simulink model "M10B39_es_V1"  (R2024b)
settings: Solver=ode23tb  StartTime=0.0  StopTime=20  FixedStep=0.001  RelTol=1e-3  EnableMultiTasking=on
InitFcn:
  | initAll;
values from neighbouring files (symbols this model uses):
  acom = 100    [initAll_V1.m]    (also in initAll_V2.m; initAll_V3.m; parameterinit.mat)
  AVm0 = [4.26082678503 4.656135219]    [parameterinit.mat]
  bcom = 50    [initAll_V1.m]    (also in initAll_V2.m; initAll_V3.m; parameterinit.mat)
  commun = 0*commun    [initAll_V1.m]    (also in initAll_V2.m; initAll_V3.m; parameterinit.mat = [0  0  0; 0  0  0; 0  0  0; 0  0  0])
  DataDelay = 0.0*DataDelay    [initAll_V1.m]    (also in initAll_V2.m; initAll_V3.m; parameterinit.mat = [0  0  0; 0  0  0; 0  0  0; 0  0  0])
  ESinit =     [parameterinit.mat]
  fB = 50    [initAll.m]    (also in initAll_V1.m; initAll_V2.m; initAll_V3.m; parameterinit.mat)
  Geninit = Generator_init(opdata,SynMach_in_gidx)    [initAll.m]    (also in initAll_V1.m; initAll_V2.m; initAll_V3.m = Generator_init(opdata_all,SynMach_in_gidx1); parameterinit.mat = )
  lam = 100    [initAll_V1.m]    (also in initAll_V2.m; initAll_V3.m; parameterinit.mat)
  SgridB = 100    [initAll.m]    (also in initAll_V1.m; initAll_V2.m; initAll_V3.m; parameterinit.mat)
  wB = 2*pi*fB    (= 314.159265359)    [initAll.m]    (also in initAll_V1.m; initAll_V2.m; initAll_V3.m; parameterinit.mat)
  Windinit =     [parameterinit.mat]
  YY_load = [3.65450097002 -2.05705688056 0 0 0 0 0 0 0 0 0 0 ... (1521 elements, 39x39)]    [parameterinit.mat]    (also in powerflowcaculate.m = full(YY))
undefined symbols (not defined in the file or in its folder): c1, c2, c3, c4, c5, c6, cp_nom, lambda_nom, P_wind_base, Pelec_base, Pnom
libraries: spsBistableLib x12, simulink_extras x4, slpidlib x1, simulink x1
(part 7 of 7)

== system M10B39_es_V1/Genrators/Wind Generator - DFIG1/Asynchronous Machine Equations /3th order Transient Equations ==
  note: Comparison of 5th order and 3rd order machine models for doubly fed induction generator (DFIG) wind turbines
      | //J.B. Ekanayake a,c, * , L. Holdsworth b , N. Jenkins b,c
  Isxy : Inport
  Vrxy : Inport  Port=2
  s / ω_B : Inport  Port=3
  Trip : Inport  Port=4
  Add : Sum  Inputs=+-
  Add1 : Sum  Inputs=-+
  Add2 : Sum  Inputs=+-
  Add3 : Sum  Inputs=--
  Constant1 : Constant  Value=0
  Constant2 : Constant  Value=0
  Demux : Demux  Outputs=2
  Demux1 : Demux  Outputs=2
  Demux2 : Demux  Outputs=2
  Ex : Integrator  InitialCondition=Ex0
  Ey : Integrator  InitialCondition=Ey0
  Fcn : Fcn  Expr=u(2)-(Xa-Xa1)*u(1)
  Fcn1 : Fcn  Expr=u(2)+(Xa-Xa1)*u(1)
  Gain{,1,6,8} (4 alike) : Gain  Gain=Lm/Lr
  Gain2 : Gain  Gain=1/Ta0
  Gain3 : Gain  Gain=1/Ta0
  Gain5 : Gain  Gain=1/Lm
  Gain7 : Gain  Gain=1/Lm
  Multiply : Product
  Multiply1 : Product  Inputs=3
  Multiply2 : Product
  Multiply3 : Product  Inputs=3
  Mux{,1..3} (4 alike) : Mux  Inputs=2
  Sum : Sum  Inputs=|+-
  Sum1 : Sum  Inputs=|+-
  Switch{1..4} (4 alike) : Switch  Criteria=u2 ~= 0  Threshold=0.5  InputSameDT=off
  Irxy : Outport
  Eyx : Outport  Port=2
  wires:
  [Trip] -> Switch4/2, Switch1/2
  Constant2/1 -> Switch4/1, Switch1/1
  Switch4/1 -> Mux/2, [Ey], Mux2/1
  Ey/1 -> Switch4/3  "Ey"
  Switch1/1 -> Ey/1
  Sum/1 -> Switch1/3
  [Trip] -> Switch2/2, Switch3/2
  Constant1/1 -> Switch3/1, Switch2/1
  Switch3/1 -> Mux1/2, [Ex], Mux2/2
  Ex/1 -> Switch3/3  "Ex"
  Sum1/1 -> Switch2/3
  Switch2/1 -> Ex/1
  Trip/1 -> [Trip]
  [Vry] -> Gain8/1
  Gain8/1 -> Multiply2/1
  Gain/1 -> Multiply/1
  Add3/1 -> [Iry]
  [Isy] -> Gain1/1
  Add2/1 -> [Irx]
  Gain1/1 -> Add3/2
  [Isx] -> Gain6/1
  [Ey] -> Gain5/1
  Gain7/1 -> Add3/1
  [Ex] -> Gain7/1
  Gain6/1 -> Add2/2
  Gain5/1 -> Add2/1
  [Irx] -> Mux3/1
  [Iry] -> Mux3/2
  Mux3/1 -> Irxy/1
  Gain2/1 -> Sum/2
  Gain3/1 -> Sum1/2
  Mux2/1 -> Eyx/1
  Fcn1/1 -> Gain3/1
  Mux1/1 -> Fcn1/1
  [Isy] -> Mux1/1
  Add1/1 -> Sum1/1
  Multiply2/1 -> Add1/1
  Multiply3/1 -> Add1/2
  [s] -> Multiply3/1
  [Ey] -> Multiply3/3
  [w_b] -> Multiply3/2
  [w_b] -> Multiply2/2
  Multiply1/1 -> Add/2
  Add/1 -> Sum/1
  Multiply/1 -> Add/1
  Fcn/1 -> Gain2/1
  Mux/1 -> Fcn/1
  [Isx] -> Mux/1
  [Ex] -> Multiply1/3
  [w_b] -> Multiply1/2
  [s] -> Multiply1/1
  [w_b] -> Multiply/2
  [Vrx] -> Gain/1
  Demux1/2 -> [Vry]
  Demux1/1 -> [Vrx]
  Demux2/2 -> [w_b]
  Demux2/1 -> [s]
  s / ω_B/1 -> Demux2/1
  Vrxy/1 -> Demux1/1
  Isxy/1 -> Demux/1
  Demux/2 -> [Isy]
  Demux/1 -> [Isx]

== system M10B39_es_V1/Genrators/Wind Generator - DFIG1/Asynchronous Machine Equations /Interface ==
  delta : Inport
  Eqd : Inport  Port=2
  Add2 : Sum
  Add3 : Sum
  Bx : Constant  Value=Xa1/( Rs^2+Xa1^2 )
  By : Constant  Value=-Xa1/( Rs^2+Xa1^2 )
  Demux1 : Demux  Outputs=2
  Fcn : Fcn  Expr=(Rs*cos(u(1))+Xa1*sin(u(1))) / (Rs^2+Xa1^2)
  Fcn1 : Fcn  Expr=(Rs*cos(u(1))+Xa1*sin(u(1))) / (Rs^2+Xa1^2)
  Fcn2 : Fcn  Expr=(-Rs*sin(u(1))+Xa1*cos(u(1))) / (Rs^2+Xa1^2)
  Fcn3 : Fcn  Expr=(Rs*sin(u(1))-Xa1*cos(u(1))) / (Rs^2+Xa1^2)
  Gx : Constant  Value=Rs/( Rs^2+Xa1^2 )
  Gy : Constant  Value=Rs/( Rs^2+Xa1^2 )
  Mux3 : Mux  Inputs=2
  Mux4 : Mux
  Product{4..7} (4 alike) : Product
  Igxy1 : Outport
  GBxy : Outport  Port=2
  wires:
  Gx/1 -> Mux4/1
  [gx] -> Product4/1
  [Eq] -> Product5/1
  Product7/1 -> Add3/2
  Product4/1 -> Add2/1
  Product5/1 -> Add2/2
  Add3/1 -> [I1y]
  Product6/1 -> Add3/1
  [Eq] -> Product7/1
  [gy] -> Product7/2
  [bx] -> Product5/2
  Add2/1 -> [I1x]
  [Ed] -> Product6/2
  [Ed] -> Product4/2
  [by] -> Product6/1
  Fcn3/1 -> [by]
  Fcn2/1 -> [bx]
  Fcn1/1 -> [gy]
  Fcn/1 -> [gx]
  [delta] -> Fcn/1, Fcn3/1, Fcn2/1, Fcn1/1
  Demux1/2 -> [Ed]
  Demux1/1 -> [Eq]
  Mux4/1 -> GBxy/1
  By/1 -> Mux4/4
  Bx/1 -> Mux4/3
  Gy/1 -> Mux4/2
  Mux3/1 -> Igxy1/1
  [I1y] -> Mux3/2
  [I1x] -> Mux3/1
  Eqd/1 -> Demux1/1
  delta/1 -> [delta]

== system M10B39_es_V1/Genrators/Wind Generator - DFIG1/Rotor Side Converter control/Power Control ==
  note: $P_s^{ref}=2*(0.5000*\omega_r^2+0.0500*\omega_r+0.1200)$
  wr : Inport
  0-inf1 : Saturate  UpperLimit=inf  LowerLimit=0
  Tracking Curve5 : Fcn  Expr=1.162*u(1)^2
  Ps_ref : Outport
  wires:
  Tracking Curve5/1 -> Ps_ref/1
  0-inf1/1 -> Tracking Curve5/1
  wr/1 -> 0-inf1/1

== system M10B39_es_V1/Genrators/Wind Generator - DFIG1/Wind Turbine/Subsystem ==
  wind speed : Inport
  generator speed : Inport  Port=2
  Pitch angle (deg) : Inport  Port=3
  1/cp_nom : Gain  Gain=1/cp_nom  SaturateOnIntegerOverflow=on  OutDataTypeStr=Inherit: Same as input  ParamDataTypeStr=Inherit: Same as input
  Avoid division by zero : Saturate  UpperLimit=1e6  LowerLimit=1e-6
  "Avoid division by zero " : Saturate  UpperLimit=1e6  LowerLimit=1e-6
  Fcn : Fcn  Expr=1/(1/(u[1]+0.08*u[2])-0.035/(u[2]^3+1))
  Fcn1 : Fcn  Expr=c1*(c2/u[2]-c3*u[3]-c4)*exp(-c5/u[2])+c6*u[1]
  Gain : Gain  Gain=-1  SaturateOnIntegerOverflow=on  OutDataTypeStr=Inherit: Same as input  ParamDataTypeStr=Inherit: Same as input
  Mux : Mux  Inputs=2
  Mux1 : Mux  Inputs=3
  Product : Product  Inputs=/*  SaturateOnIntegerOverflow=on  OutDataTypeStr=Inherit: Same as first input
  "Product " : Product  SaturateOnIntegerOverflow=on  OutDataTypeStr=Inherit: Same as first input
  Product1 : Product  Inputs=*/  InputSameDT=on  SaturateOnIntegerOverflow=on  OutDataTypeStr=Inherit: Same as first input
  Saturation1 : Saturate  UpperLimit=inf  LowerLimit=1e-6
  lambda_nom : Gain  Gain=lambda_nom  SaturateOnIntegerOverflow=on  OutDataTypeStr=Inherit: Same as input  ParamDataTypeStr=Inherit: Same as input
  pu->pu : Gain  Gain=P_wind_base*Pnom/Pelec_base  SaturateOnIntegerOverflow=on  OutDataTypeStr=Inherit: Same as input  ParamDataTypeStr=Inherit: Same as input
  wind_speed^3 : Fcn  Expr=u(1)^3
  Tm : Outport
  wires:
  Pitch angle (deg)/1 -> Mux/2, Mux1/3
  Saturation1/1 -> Mux/1, Mux1/1
  Fcn1/1 -> 1/cp_nom/1
  Mux1/1 -> Fcn1/1
  Mux/1 -> Fcn/1
  Fcn/1 -> Mux1/2  "lambda_i"
  Gain/1 -> Tm/1
  Product1/1 -> Gain/1
  "Product "/1 -> pu->pu/1  "Pm_pu"
  lambda_nom/1 -> Saturation1/1
  generator speed/1 -> Avoid division by zero/1, Product/2
  "Avoid division by zero "/1 -> Product/1
  pu->pu/1 -> Product1/1
  Product/1 -> lambda_nom/1
  Avoid division by zero/1 -> Product1/2
  wind_speed^3/1 -> "Product "/1  "Pwind_pu"
  1/cp_nom/1 -> "Product "/2  "cp_pu"
  wind speed/1 -> "Avoid division by zero "/1, wind_speed^3/1  "wind_speed_pu"

== system M10B39_es_V1/Genrators/Wind Generator - DFIG2/Asynchronous Machine Equations /3th order Transient Equations ==
  note: Comparison of 5th order and 3rd order machine models for doubly fed induction generator (DFIG) wind turbines
      | //J.B. Ekanayake a,c, * , L. Holdsworth b , N. Jenkins b,c
  Isxy : Inport
  Vrxy : Inport  Port=2
  s / ω_B : Inport  Port=3
  Trip : Inport  Port=4
  Add : Sum  Inputs=+-
  Add1 : Sum  Inputs=-+
  Add2 : Sum  Inputs=+-
  Add3 : Sum  Inputs=--
  Constant1 : Constant  Value=0
  Constant2 : Constant  Value=0
  Demux : Demux  Outputs=2
  Demux1 : Demux  Outputs=2
  Demux2 : Demux  Outputs=2
  Ex : Integrator  InitialCondition=Ex0
  Ey : Integrator  InitialCondition=Ey0
  Fcn : Fcn  Expr=u(2)-(Xa-Xa1)*u(1)
  Fcn1 : Fcn  Expr=u(2)+(Xa-Xa1)*u(1)
  Gain{,1,6,8} (4 alike) : Gain  Gain=Lm/Lr
  Gain2 : Gain  Gain=1/Ta0
  Gain3 : Gain  Gain=1/Ta0
  Gain5 : Gain  Gain=1/Lm
  Gain7 : Gain  Gain=1/Lm
  Multiply : Product
  Multiply1 : Product  Inputs=3
  Multiply2 : Product
  Multiply3 : Product  Inputs=3
  Mux{,1..3} (4 alike) : Mux  Inputs=2
  Sum : Sum  Inputs=|+-
  Sum1 : Sum  Inputs=|+-
  Switch{1..4} (4 alike) : Switch  Criteria=u2 ~= 0  Threshold=0.5  InputSameDT=off
  Irxy : Outport
  Eyx : Outport  Port=2
  wires:
  [Trip] -> Switch4/2, Switch1/2
  Constant2/1 -> Switch4/1, Switch1/1
  Switch4/1 -> Mux/2, [Ey], Mux2/1
  Ey/1 -> Switch4/3  "Ey"
  Switch1/1 -> Ey/1
  Sum/1 -> Switch1/3
  [Trip] -> Switch2/2, Switch3/2
  Constant1/1 -> Switch3/1, Switch2/1
  Switch3/1 -> Mux1/2, [Ex], Mux2/2
  Ex/1 -> Switch3/3  "Ex"
  Sum1/1 -> Switch2/3
  Switch2/1 -> Ex/1
  Trip/1 -> [Trip]
  [Vry] -> Gain8/1
  Gain8/1 -> Multiply2/1
  Gain/1 -> Multiply/1
  Add3/1 -> [Iry]
  [Isy] -> Gain1/1
  Add2/1 -> [Irx]
  Gain1/1 -> Add3/2
  [Isx] -> Gain6/1
  [Ey] -> Gain5/1
  Gain7/1 -> Add3/1
  [Ex] -> Gain7/1
  Gain6/1 -> Add2/2
  Gain5/1 -> Add2/1
  [Irx] -> Mux3/1
  [Iry] -> Mux3/2
  Mux3/1 -> Irxy/1
  Gain2/1 -> Sum/2
  Gain3/1 -> Sum1/2
  Mux2/1 -> Eyx/1
  Fcn1/1 -> Gain3/1
  Mux1/1 -> Fcn1/1
  [Isy] -> Mux1/1
  Add1/1 -> Sum1/1
  Multiply2/1 -> Add1/1
  Multiply3/1 -> Add1/2
  [s] -> Multiply3/1
  [Ey] -> Multiply3/3
  [w_b] -> Multiply3/2
  [w_b] -> Multiply2/2
  Multiply1/1 -> Add/2
  Add/1 -> Sum/1
  Multiply/1 -> Add/1
  Fcn/1 -> Gain2/1
  Mux/1 -> Fcn/1
  [Isx] -> Mux/1
  [Ex] -> Multiply1/3
  [w_b] -> Multiply1/2
  [s] -> Multiply1/1
  [w_b] -> Multiply/2
  [Vrx] -> Gain/1
  Demux1/2 -> [Vry]
  Demux1/1 -> [Vrx]
  Demux2/2 -> [w_b]
  Demux2/1 -> [s]
  s / ω_B/1 -> Demux2/1
  Vrxy/1 -> Demux1/1
  Isxy/1 -> Demux/1
  Demux/2 -> [Isy]
  Demux/1 -> [Isx]

== system M10B39_es_V1/Genrators/Wind Generator - DFIG2/Asynchronous Machine Equations /Interface ==
  delta : Inport
  Eqd : Inport  Port=2
  Add2 : Sum
  Add3 : Sum
  Bx : Constant  Value=Xa1/( Rs^2+Xa1^2 )
  By : Constant  Value=-Xa1/( Rs^2+Xa1^2 )
  Demux1 : Demux  Outputs=2
  Fcn : Fcn  Expr=(Rs*cos(u(1))+Xa1*sin(u(1))) / (Rs^2+Xa1^2)
  Fcn1 : Fcn  Expr=(Rs*cos(u(1))+Xa1*sin(u(1))) / (Rs^2+Xa1^2)
  Fcn2 : Fcn  Expr=(-Rs*sin(u(1))+Xa1*cos(u(1))) / (Rs^2+Xa1^2)
  Fcn3 : Fcn  Expr=(Rs*sin(u(1))-Xa1*cos(u(1))) / (Rs^2+Xa1^2)
  Gx : Constant  Value=Rs/( Rs^2+Xa1^2 )
  Gy : Constant  Value=Rs/( Rs^2+Xa1^2 )
  Mux3 : Mux  Inputs=2
  Mux4 : Mux
  Product{4..7} (4 alike) : Product
  Igxy1 : Outport
  GBxy : Outport  Port=2
  wires:
  Gx/1 -> Mux4/1
  [gx] -> Product4/1
  [Eq] -> Product5/1
  Product7/1 -> Add3/2
  Product4/1 -> Add2/1
  Product5/1 -> Add2/2
  Add3/1 -> [I1y]
  Product6/1 -> Add3/1
  [Eq] -> Product7/1
  [gy] -> Product7/2
  [bx] -> Product5/2
  Add2/1 -> [I1x]
  [Ed] -> Product6/2
  [Ed] -> Product4/2
  [by] -> Product6/1
  Fcn3/1 -> [by]
  Fcn2/1 -> [bx]
  Fcn1/1 -> [gy]
  Fcn/1 -> [gx]
  [delta] -> Fcn/1, Fcn3/1, Fcn2/1, Fcn1/1
  Demux1/2 -> [Ed]
  Demux1/1 -> [Eq]
  Mux4/1 -> GBxy/1
  By/1 -> Mux4/4
  Bx/1 -> Mux4/3
  Gy/1 -> Mux4/2
  Mux3/1 -> Igxy1/1
  [I1y] -> Mux3/2
  [I1x] -> Mux3/1
  Eqd/1 -> Demux1/1
  delta/1 -> [delta]

== system M10B39_es_V1/Genrators/Wind Generator - DFIG2/Rotor Side Converter control/Power Control ==
  note: $P_s^{ref}=2*(0.5000*\omega_r^2+0.0500*\omega_r+0.1200)$
  wr : Inport
  0-inf1 : Saturate  UpperLimit=inf  LowerLimit=0
  Tracking Curve5 : Fcn  Expr=1.162*u(1)^2
  Ps_ref : Outport
  wires:
  Tracking Curve5/1 -> Ps_ref/1
  0-inf1/1 -> Tracking Curve5/1
  wr/1 -> 0-inf1/1

== system M10B39_es_V1/Genrators/Wind Generator - DFIG2/Wind Turbine/Subsystem ==
  wind speed : Inport
  generator speed : Inport  Port=2
  Pitch angle (deg) : Inport  Port=3
  1/cp_nom : Gain  Gain=1/cp_nom  SaturateOnIntegerOverflow=on  OutDataTypeStr=Inherit: Same as input  ParamDataTypeStr=Inherit: Same as input
  Avoid division by zero : Saturate  UpperLimit=1e6  LowerLimit=1e-6
  "Avoid division by zero " : Saturate  UpperLimit=1e6  LowerLimit=1e-6
  Fcn : Fcn  Expr=1/(1/(u[1]+0.08*u[2])-0.035/(u[2]^3+1))
  Fcn1 : Fcn  Expr=c1*(c2/u[2]-c3*u[3]-c4)*exp(-c5/u[2])+c6*u[1]
  Gain : Gain  Gain=-1  SaturateOnIntegerOverflow=on  OutDataTypeStr=Inherit: Same as input  ParamDataTypeStr=Inherit: Same as input
  Mux : Mux  Inputs=2
  Mux1 : Mux  Inputs=3
  Product : Product  Inputs=/*  SaturateOnIntegerOverflow=on  OutDataTypeStr=Inherit: Same as first input
  "Product " : Product  SaturateOnIntegerOverflow=on  OutDataTypeStr=Inherit: Same as first input
  Product1 : Product  Inputs=*/  InputSameDT=on  SaturateOnIntegerOverflow=on  OutDataTypeStr=Inherit: Same as first input
  Saturation1 : Saturate  UpperLimit=inf  LowerLimit=1e-6
  lambda_nom : Gain  Gain=lambda_nom  SaturateOnIntegerOverflow=on  OutDataTypeStr=Inherit: Same as input  ParamDataTypeStr=Inherit: Same as input
  pu->pu : Gain  Gain=P_wind_base*Pnom/Pelec_base  SaturateOnIntegerOverflow=on  OutDataTypeStr=Inherit: Same as input  ParamDataTypeStr=Inherit: Same as input
  wind_speed^3 : Fcn  Expr=u(1)^3
  Tm : Outport
  wires:
  Pitch angle (deg)/1 -> Mux/2, Mux1/3
  Saturation1/1 -> Mux/1, Mux1/1
  Fcn1/1 -> 1/cp_nom/1
  Mux1/1 -> Fcn1/1
  Mux/1 -> Fcn/1
  Fcn/1 -> Mux1/2  "lambda_i"
  Gain/1 -> Tm/1
  Product1/1 -> Gain/1
  "Product "/1 -> pu->pu/1  "Pm_pu"
  lambda_nom/1 -> Saturation1/1
  generator speed/1 -> Avoid division by zero/1, Product/2
  "Avoid division by zero "/1 -> Product/1
  pu->pu/1 -> Product1/1
  Product/1 -> lambda_nom/1
  Avoid division by zero/1 -> Product1/2
  wind_speed^3/1 -> "Product "/1  "Pwind_pu"
  1/cp_nom/1 -> "Product "/2  "cp_pu"
  wind speed/1 -> "Avoid division by zero "/1, wind_speed^3/1  "wind_speed_pu"

== system M10B39_es_V1/Genrators/Wind Generator - DFIG3/Asynchronous Machine Equations /3th order Transient Equations ==
  note: Comparison of 5th order and 3rd order machine models for doubly fed induction generator (DFIG) wind turbines
      | //J.B. Ekanayake a,c, * , L. Holdsworth b , N. Jenkins b,c
  Isxy : Inport
  Vrxy : Inport  Port=2
  s / ω_B : Inport  Port=3
  Trip : Inport  Port=4
  Add : Sum  Inputs=+-
  Add1 : Sum  Inputs=-+
  Add2 : Sum  Inputs=+-
  Add3 : Sum  Inputs=--
  Constant1 : Constant  Value=0
  Constant2 : Constant  Value=0
  Demux : Demux  Outputs=2
  Demux1 : Demux  Outputs=2
  Demux2 : Demux  Outputs=2
  Ex : Integrator  InitialCondition=Ex0
  Ey : Integrator  InitialCondition=Ey0
  Fcn : Fcn  Expr=u(2)-(Xa-Xa1)*u(1)
  Fcn1 : Fcn  Expr=u(2)+(Xa-Xa1)*u(1)
  Gain{,1,6,8} (4 alike) : Gain  Gain=Lm/Lr
  Gain2 : Gain  Gain=1/Ta0
  Gain3 : Gain  Gain=1/Ta0
  Gain5 : Gain  Gain=1/Lm
  Gain7 : Gain  Gain=1/Lm
  Multiply : Product
  Multiply1 : Product  Inputs=3
  Multiply2 : Product
  Multiply3 : Product  Inputs=3
  Mux{,1..3} (4 alike) : Mux  Inputs=2
  Sum : Sum  Inputs=|+-
  Sum1 : Sum  Inputs=|+-
  Switch{1..4} (4 alike) : Switch  Criteria=u2 ~= 0  Threshold=0.5  InputSameDT=off
  Irxy : Outport
  Eyx : Outport  Port=2
  wires:
  [Trip] -> Switch4/2, Switch1/2
  Constant2/1 -> Switch4/1, Switch1/1
  Switch4/1 -> Mux/2, [Ey], Mux2/1
  Ey/1 -> Switch4/3  "Ey"
  Switch1/1 -> Ey/1
  Sum/1 -> Switch1/3
  [Trip] -> Switch2/2, Switch3/2
  Constant1/1 -> Switch3/1, Switch2/1
  Switch3/1 -> Mux1/2, [Ex], Mux2/2
  Ex/1 -> Switch3/3  "Ex"
  Sum1/1 -> Switch2/3
  Switch2/1 -> Ex/1
  Trip/1 -> [Trip]
  [Vry] -> Gain8/1
  Gain8/1 -> Multiply2/1
  Gain/1 -> Multiply/1
  Add3/1 -> [Iry]
  [Isy] -> Gain1/1
  Add2/1 -> [Irx]
  Gain1/1 -> Add3/2
  [Isx] -> Gain6/1
  [Ey] -> Gain5/1
  Gain7/1 -> Add3/1
  [Ex] -> Gain7/1
  Gain6/1 -> Add2/2
  Gain5/1 -> Add2/1
  [Irx] -> Mux3/1
  [Iry] -> Mux3/2
  Mux3/1 -> Irxy/1
  Gain2/1 -> Sum/2
  Gain3/1 -> Sum1/2
  Mux2/1 -> Eyx/1
  Fcn1/1 -> Gain3/1
  Mux1/1 -> Fcn1/1
  [Isy] -> Mux1/1
  Add1/1 -> Sum1/1
  Multiply2/1 -> Add1/1
  Multiply3/1 -> Add1/2
  [s] -> Multiply3/1
  [Ey] -> Multiply3/3
  [w_b] -> Multiply3/2
  [w_b] -> Multiply2/2
  Multiply1/1 -> Add/2
  Add/1 -> Sum/1
  Multiply/1 -> Add/1
  Fcn/1 -> Gain2/1
  Mux/1 -> Fcn/1
  [Isx] -> Mux/1
  [Ex] -> Multiply1/3
  [w_b] -> Multiply1/2
  [s] -> Multiply1/1
  [w_b] -> Multiply/2
  [Vrx] -> Gain/1
  Demux1/2 -> [Vry]
  Demux1/1 -> [Vrx]
  Demux2/2 -> [w_b]
  Demux2/1 -> [s]
  s / ω_B/1 -> Demux2/1
  Vrxy/1 -> Demux1/1
  Isxy/1 -> Demux/1
  Demux/2 -> [Isy]
  Demux/1 -> [Isx]

== system M10B39_es_V1/Genrators/Wind Generator - DFIG3/Asynchronous Machine Equations /Interface ==
  delta : Inport
  Eqd : Inport  Port=2
  Add2 : Sum
  Add3 : Sum
  Bx : Constant  Value=Xa1/( Rs^2+Xa1^2 )
  By : Constant  Value=-Xa1/( Rs^2+Xa1^2 )
  Demux1 : Demux  Outputs=2
  Fcn : Fcn  Expr=(Rs*cos(u(1))+Xa1*sin(u(1))) / (Rs^2+Xa1^2)
  Fcn1 : Fcn  Expr=(Rs*cos(u(1))+Xa1*sin(u(1))) / (Rs^2+Xa1^2)
  Fcn2 : Fcn  Expr=(-Rs*sin(u(1))+Xa1*cos(u(1))) / (Rs^2+Xa1^2)
  Fcn3 : Fcn  Expr=(Rs*sin(u(1))-Xa1*cos(u(1))) / (Rs^2+Xa1^2)
  Gx : Constant  Value=Rs/( Rs^2+Xa1^2 )
  Gy : Constant  Value=Rs/( Rs^2+Xa1^2 )
  Mux3 : Mux  Inputs=2
  Mux4 : Mux
  Product{4..7} (4 alike) : Product
  Igxy1 : Outport
  GBxy : Outport  Port=2
  wires:
  Gx/1 -> Mux4/1
  [gx] -> Product4/1
  [Eq] -> Product5/1
  Product7/1 -> Add3/2
  Product4/1 -> Add2/1
  Product5/1 -> Add2/2
  Add3/1 -> [I1y]
  Product6/1 -> Add3/1
  [Eq] -> Product7/1
  [gy] -> Product7/2
  [bx] -> Product5/2
  Add2/1 -> [I1x]
  [Ed] -> Product6/2
  [Ed] -> Product4/2
  [by] -> Product6/1
  Fcn3/1 -> [by]
  Fcn2/1 -> [bx]
  Fcn1/1 -> [gy]
  Fcn/1 -> [gx]
  [delta] -> Fcn/1, Fcn3/1, Fcn2/1, Fcn1/1
  Demux1/2 -> [Ed]
  Demux1/1 -> [Eq]
  Mux4/1 -> GBxy/1
  By/1 -> Mux4/4
  Bx/1 -> Mux4/3
  Gy/1 -> Mux4/2
  Mux3/1 -> Igxy1/1
  [I1y] -> Mux3/2
  [I1x] -> Mux3/1
  Eqd/1 -> Demux1/1
  delta/1 -> [delta]

== system M10B39_es_V1/Genrators/Wind Generator - DFIG3/Rotor Side Converter control/Power Control ==
  note: $P_s^{ref}=2*(0.5000*\omega_r^2+0.0500*\omega_r+0.1200)$
  wr : Inport
  0-inf1 : Saturate  UpperLimit=inf  LowerLimit=0
  Tracking Curve5 : Fcn  Expr=1.162*u(1)^2
  Ps_ref : Outport
  wires:
  Tracking Curve5/1 -> Ps_ref/1
  0-inf1/1 -> Tracking Curve5/1
  wr/1 -> 0-inf1/1

== system M10B39_es_V1/Genrators/Wind Generator - DFIG3/Wind Turbine/Subsystem ==
  wind speed : Inport
  generator speed : Inport  Port=2
  Pitch angle (deg) : Inport  Port=3
  1/cp_nom : Gain  Gain=1/cp_nom  SaturateOnIntegerOverflow=on  OutDataTypeStr=Inherit: Same as input  ParamDataTypeStr=Inherit: Same as input
  Avoid division by zero : Saturate  UpperLimit=1e6  LowerLimit=1e-6
  "Avoid division by zero " : Saturate  UpperLimit=1e6  LowerLimit=1e-6
  Fcn : Fcn  Expr=1/(1/(u[1]+0.08*u[2])-0.035/(u[2]^3+1))
  Fcn1 : Fcn  Expr=c1*(c2/u[2]-c3*u[3]-c4)*exp(-c5/u[2])+c6*u[1]
  Gain : Gain  Gain=-1  SaturateOnIntegerOverflow=on  OutDataTypeStr=Inherit: Same as input  ParamDataTypeStr=Inherit: Same as input
  Mux : Mux  Inputs=2
  Mux1 : Mux  Inputs=3
  Product : Product  Inputs=/*  SaturateOnIntegerOverflow=on  OutDataTypeStr=Inherit: Same as first input
  "Product " : Product  SaturateOnIntegerOverflow=on  OutDataTypeStr=Inherit: Same as first input
  Product1 : Product  Inputs=*/  InputSameDT=on  SaturateOnIntegerOverflow=on  OutDataTypeStr=Inherit: Same as first input
  Saturation1 : Saturate  UpperLimit=inf  LowerLimit=1e-6
  lambda_nom : Gain  Gain=lambda_nom  SaturateOnIntegerOverflow=on  OutDataTypeStr=Inherit: Same as input  ParamDataTypeStr=Inherit: Same as input
  pu->pu : Gain  Gain=P_wind_base*Pnom/Pelec_base  SaturateOnIntegerOverflow=on  OutDataTypeStr=Inherit: Same as input  ParamDataTypeStr=Inherit: Same as input
  wind_speed^3 : Fcn  Expr=u(1)^3
  Tm : Outport
  wires:
  Pitch angle (deg)/1 -> Mux/2, Mux1/3
  Saturation1/1 -> Mux/1, Mux1/1
  Fcn1/1 -> 1/cp_nom/1
  Mux1/1 -> Fcn1/1
  Mux/1 -> Fcn/1
  Fcn/1 -> Mux1/2  "lambda_i"
  Gain/1 -> Tm/1
  Product1/1 -> Gain/1
  "Product "/1 -> pu->pu/1  "Pm_pu"
  lambda_nom/1 -> Saturation1/1
  generator speed/1 -> Avoid division by zero/1, Product/2
  "Avoid division by zero "/1 -> Product/1
  pu->pu/1 -> Product1/1
  Product/1 -> lambda_nom/1
  Avoid division by zero/1 -> Product1/2
  wind_speed^3/1 -> "Product "/1  "Pwind_pu"
  1/cp_nom/1 -> "Product "/2  "cp_pu"
  wind speed/1 -> "Avoid division by zero "/1, wind_speed^3/1  "wind_speed_pu"

== system M10B39_es_V1/Genrators/Wind Generator - DFIG4/Asynchronous Machine Equations /3th order Transient Equations ==
  note: Comparison of 5th order and 3rd order machine models for doubly fed induction generator (DFIG) wind turbines
      | //J.B. Ekanayake a,c, * , L. Holdsworth b , N. Jenkins b,c
  Isxy : Inport
  Vrxy : Inport  Port=2
  s / ω_B : Inport  Port=3
  Trip : Inport  Port=4
  Add : Sum  Inputs=+-
  Add1 : Sum  Inputs=-+
  Add2 : Sum  Inputs=+-
  Add3 : Sum  Inputs=--
  Constant1 : Constant  Value=0
  Constant2 : Constant  Value=0
  Demux : Demux  Outputs=2
  Demux1 : Demux  Outputs=2
  Demux2 : Demux  Outputs=2
  Ex : Integrator  InitialCondition=Ex0
  Ey : Integrator  InitialCondition=Ey0
  Fcn : Fcn  Expr=u(2)-(Xa-Xa1)*u(1)
  Fcn1 : Fcn  Expr=u(2)+(Xa-Xa1)*u(1)
  Gain{,1,6,8} (4 alike) : Gain  Gain=Lm/Lr
  Gain2 : Gain  Gain=1/Ta0
  Gain3 : Gain  Gain=1/Ta0
  Gain5 : Gain  Gain=1/Lm
  Gain7 : Gain  Gain=1/Lm
  Multiply : Product
  Multiply1 : Product  Inputs=3
  Multiply2 : Product
  Multiply3 : Product  Inputs=3
  Mux{,1..3} (4 alike) : Mux  Inputs=2
  Sum : Sum  Inputs=|+-
  Sum1 : Sum  Inputs=|+-
  Switch{1..4} (4 alike) : Switch  Criteria=u2 ~= 0  Threshold=0.5  InputSameDT=off
  Irxy : Outport
  Eyx : Outport  Port=2
  wires:
  [Trip] -> Switch4/2, Switch1/2
  Constant2/1 -> Switch4/1, Switch1/1
  Switch4/1 -> Mux/2, [Ey], Mux2/1
  Ey/1 -> Switch4/3  "Ey"
  Switch1/1 -> Ey/1
  Sum/1 -> Switch1/3
  [Trip] -> Switch2/2, Switch3/2
  Constant1/1 -> Switch3/1, Switch2/1
  Switch3/1 -> Mux1/2, [Ex], Mux2/2
  Ex/1 -> Switch3/3  "Ex"
  Sum1/1 -> Switch2/3
  Switch2/1 -> Ex/1
  Trip/1 -> [Trip]
  [Vry] -> Gain8/1
  Gain8/1 -> Multiply2/1
  Gain/1 -> Multiply/1
  Add3/1 -> [Iry]
  [Isy] -> Gain1/1
  Add2/1 -> [Irx]
  Gain1/1 -> Add3/2
  [Isx] -> Gain6/1
  [Ey] -> Gain5/1
  Gain7/1 -> Add3/1
  [Ex] -> Gain7/1
  Gain6/1 -> Add2/2
  Gain5/1 -> Add2/1
  [Irx] -> Mux3/1
  [Iry] -> Mux3/2
  Mux3/1 -> Irxy/1
  Gain2/1 -> Sum/2
  Gain3/1 -> Sum1/2
  Mux2/1 -> Eyx/1
  Fcn1/1 -> Gain3/1
  Mux1/1 -> Fcn1/1
  [Isy] -> Mux1/1
  Add1/1 -> Sum1/1
  Multiply2/1 -> Add1/1
  Multiply3/1 -> Add1/2
  [s] -> Multiply3/1
  [Ey] -> Multiply3/3
  [w_b] -> Multiply3/2
  [w_b] -> Multiply2/2
  Multiply1/1 -> Add/2
  Add/1 -> Sum/1
  Multiply/1 -> Add/1
  Fcn/1 -> Gain2/1
  Mux/1 -> Fcn/1
  [Isx] -> Mux/1
  [Ex] -> Multiply1/3
  [w_b] -> Multiply1/2
  [s] -> Multiply1/1
  [w_b] -> Multiply/2
  [Vrx] -> Gain/1
  Demux1/2 -> [Vry]
  Demux1/1 -> [Vrx]
  Demux2/2 -> [w_b]
  Demux2/1 -> [s]
  s / ω_B/1 -> Demux2/1
  Vrxy/1 -> Demux1/1
  Isxy/1 -> Demux/1
  Demux/2 -> [Isy]
  Demux/1 -> [Isx]

== system M10B39_es_V1/Genrators/Wind Generator - DFIG4/Asynchronous Machine Equations /Interface ==
  delta : Inport
  Eqd : Inport  Port=2
  Add2 : Sum
  Add3 : Sum
  Bx : Constant  Value=Xa1/( Rs^2+Xa1^2 )
  By : Constant  Value=-Xa1/( Rs^2+Xa1^2 )
  Demux1 : Demux  Outputs=2
  Fcn : Fcn  Expr=(Rs*cos(u(1))+Xa1*sin(u(1))) / (Rs^2+Xa1^2)
  Fcn1 : Fcn  Expr=(Rs*cos(u(1))+Xa1*sin(u(1))) / (Rs^2+Xa1^2)
  Fcn2 : Fcn  Expr=(-Rs*sin(u(1))+Xa1*cos(u(1))) / (Rs^2+Xa1^2)
  Fcn3 : Fcn  Expr=(Rs*sin(u(1))-Xa1*cos(u(1))) / (Rs^2+Xa1^2)
  Gx : Constant  Value=Rs/( Rs^2+Xa1^2 )
  Gy : Constant  Value=Rs/( Rs^2+Xa1^2 )
  Mux3 : Mux  Inputs=2
  Mux4 : Mux
  Product{4..7} (4 alike) : Product
  Igxy1 : Outport
  GBxy : Outport  Port=2
  wires:
  Gx/1 -> Mux4/1
  [gx] -> Product4/1
  [Eq] -> Product5/1
  Product7/1 -> Add3/2
  Product4/1 -> Add2/1
  Product5/1 -> Add2/2
  Add3/1 -> [I1y]
  Product6/1 -> Add3/1
  [Eq] -> Product7/1
  [gy] -> Product7/2
  [bx] -> Product5/2
  Add2/1 -> [I1x]
  [Ed] -> Product6/2
  [Ed] -> Product4/2
  [by] -> Product6/1
  Fcn3/1 -> [by]
  Fcn2/1 -> [bx]
  Fcn1/1 -> [gy]
  Fcn/1 -> [gx]
  [delta] -> Fcn/1, Fcn3/1, Fcn2/1, Fcn1/1
  Demux1/2 -> [Ed]
  Demux1/1 -> [Eq]
  Mux4/1 -> GBxy/1
  By/1 -> Mux4/4
  Bx/1 -> Mux4/3
  Gy/1 -> Mux4/2
  Mux3/1 -> Igxy1/1
  [I1y] -> Mux3/2
  [I1x] -> Mux3/1
  Eqd/1 -> Demux1/1
  delta/1 -> [delta]

== system M10B39_es_V1/Genrators/Wind Generator - DFIG4/Rotor Side Converter control/Power Control ==
  note: $P_s^{ref}=2*(0.5000*\omega_r^2+0.0500*\omega_r+0.1200)$
  wr : Inport
  0-inf1 : Saturate  UpperLimit=inf  LowerLimit=0
  Tracking Curve5 : Fcn  Expr=1.162*u(1)^2
  Ps_ref : Outport
  wires:
  Tracking Curve5/1 -> Ps_ref/1
  0-inf1/1 -> Tracking Curve5/1
  wr/1 -> 0-inf1/1

== system M10B39_es_V1/Genrators/Wind Generator - DFIG4/Wind Turbine/Subsystem ==
  wind speed : Inport
  generator speed : Inport  Port=2
  Pitch angle (deg) : Inport  Port=3
  1/cp_nom : Gain  Gain=1/cp_nom  SaturateOnIntegerOverflow=on  OutDataTypeStr=Inherit: Same as input  ParamDataTypeStr=Inherit: Same as input
  Avoid division by zero : Saturate  UpperLimit=1e6  LowerLimit=1e-6
  "Avoid division by zero " : Saturate  UpperLimit=1e6  LowerLimit=1e-6
  Fcn : Fcn  Expr=1/(1/(u[1]+0.08*u[2])-0.035/(u[2]^3+1))
  Fcn1 : Fcn  Expr=c1*(c2/u[2]-c3*u[3]-c4)*exp(-c5/u[2])+c6*u[1]
  Gain : Gain  Gain=-1  SaturateOnIntegerOverflow=on  OutDataTypeStr=Inherit: Same as input  ParamDataTypeStr=Inherit: Same as input
  Mux : Mux  Inputs=2
  Mux1 : Mux  Inputs=3
  Product : Product  Inputs=/*  SaturateOnIntegerOverflow=on  OutDataTypeStr=Inherit: Same as first input
  "Product " : Product  SaturateOnIntegerOverflow=on  OutDataTypeStr=Inherit: Same as first input
  Product1 : Product  Inputs=*/  InputSameDT=on  SaturateOnIntegerOverflow=on  OutDataTypeStr=Inherit: Same as first input
  Saturation1 : Saturate  UpperLimit=inf  LowerLimit=1e-6
  lambda_nom : Gain  Gain=lambda_nom  SaturateOnIntegerOverflow=on  OutDataTypeStr=Inherit: Same as input  ParamDataTypeStr=Inherit: Same as input
  pu->pu : Gain  Gain=P_wind_base*Pnom/Pelec_base  SaturateOnIntegerOverflow=on  OutDataTypeStr=Inherit: Same as input  ParamDataTypeStr=Inherit: Same as input
  wind_speed^3 : Fcn  Expr=u(1)^3
  Tm : Outport
  wires:
  Pitch angle (deg)/1 -> Mux/2, Mux1/3
  Saturation1/1 -> Mux/1, Mux1/1
  Fcn1/1 -> 1/cp_nom/1
  Mux1/1 -> Fcn1/1
  Mux/1 -> Fcn/1
  Fcn/1 -> Mux1/2  "lambda_i"
  Gain/1 -> Tm/1
  Product1/1 -> Gain/1
  "Product "/1 -> pu->pu/1  "Pm_pu"
  lambda_nom/1 -> Saturation1/1
  generator speed/1 -> Avoid division by zero/1, Product/2
  "Avoid division by zero "/1 -> Product/1
  pu->pu/1 -> Product1/1
  Product/1 -> lambda_nom/1
  Avoid division by zero/1 -> Product1/2
  wind_speed^3/1 -> "Product "/1  "Pwind_pu"
  1/cp_nom/1 -> "Product "/2  "cp_pu"
  wind speed/1 -> "Avoid division by zero "/1, wind_speed^3/1  "wind_speed_pu"

== system M10B39_es_V1/Genrators/ES1/ control1/control_AC_voltage/Out_Q_Uac ==
  In1 : Inport
  Ki : Gain  Gain=KI_  SaturateOnIntegerOverflow=on  OutDataTypeStr=Inherit: Same as input  ParamDataTypeStr=Inherit: Same as input
  Kp : Gain  Gain=KP_  SaturateOnIntegerOverflow=on  OutDataTypeStr=Inherit: Same as input  ParamDataTypeStr=Inherit: Same as input
  Saturation2 : Saturate  UpperLimit=Upper_limit  LowerLimit=Lower_limit
  Sum12 : Sum  SaturateOnIntegerOverflow=on
  integrator : Integrator  InitialCondition=integrator_init  LimitOutput=on  UpperSaturationLimit=Upper_saturation_limit  LowerSaturationLimit=Lower_saturation_limit
  Out1 : Outport
  wires:
  In1/1 -> Ki/1, Kp/1
  Kp/1 -> Sum12/2
  Ki/1 -> integrator/1
  integrator/1 -> Sum12/1
  Saturation2/1 -> Out1/1
  Sum12/1 -> Saturation2/1

== system M10B39_es_V1/Genrators/ES1/ control1/control_AC_voltage1/Out_Q_Uac ==
  In1 : Inport
  Ki : Gain  Gain=KI_  SaturateOnIntegerOverflow=on  OutDataTypeStr=Inherit: Same as input  ParamDataTypeStr=Inherit: Same as input
  Kp : Gain  Gain=KP_  SaturateOnIntegerOverflow=on  OutDataTypeStr=Inherit: Same as input  ParamDataTypeStr=Inherit: Same as input
  Saturation2 : Saturate  UpperLimit=Upper_limit  LowerLimit=Lower_limit
  Sum12 : Sum  SaturateOnIntegerOverflow=on
  integrator : Integrator  InitialCondition=integrator_init  LimitOutput=on  UpperSaturationLimit=Upper_saturation_limit  LowerSaturationLimit=Lower_saturation_limit
  Out1 : Outport
  wires:
  In1/1 -> Ki/1, Kp/1
  Kp/1 -> Sum12/2
  Ki/1 -> integrator/1
  integrator/1 -> Sum12/1
  Saturation2/1 -> Out1/1
  Sum12/1 -> Saturation2/1

== system M10B39_es_V1/Genrators/ES2/ control1/control_AC_voltage/Out_Q_Uac ==
  In1 : Inport
  Ki : Gain  Gain=KI_  SaturateOnIntegerOverflow=on  OutDataTypeStr=Inherit: Same as input  ParamDataTypeStr=Inherit: Same as input
  Kp : Gain  Gain=KP_  SaturateOnIntegerOverflow=on  OutDataTypeStr=Inherit: Same as input  ParamDataTypeStr=Inherit: Same as input
  Saturation2 : Saturate  UpperLimit=Upper_limit  LowerLimit=Lower_limit
  Sum12 : Sum  SaturateOnIntegerOverflow=on
  integrator : Integrator  InitialCondition=integrator_init  LimitOutput=on  UpperSaturationLimit=Upper_saturation_limit  LowerSaturationLimit=Lower_saturation_limit
  Out1 : Outport
  wires:
  In1/1 -> Ki/1, Kp/1
  Kp/1 -> Sum12/2
  Ki/1 -> integrator/1
  integrator/1 -> Sum12/1
  Saturation2/1 -> Out1/1
  Sum12/1 -> Saturation2/1

== system M10B39_es_V1/Genrators/ES2/ control1/control_AC_voltage1/Out_Q_Uac ==
  In1 : Inport
  Ki : Gain  Gain=KI_  SaturateOnIntegerOverflow=on  OutDataTypeStr=Inherit: Same as input  ParamDataTypeStr=Inherit: Same as input
  Kp : Gain  Gain=KP_  SaturateOnIntegerOverflow=on  OutDataTypeStr=Inherit: Same as input  ParamDataTypeStr=Inherit: Same as input
  Saturation2 : Saturate  UpperLimit=Upper_limit  LowerLimit=Lower_limit
  Sum12 : Sum  SaturateOnIntegerOverflow=on
  integrator : Integrator  InitialCondition=integrator_init  LimitOutput=on  UpperSaturationLimit=Upper_saturation_limit  LowerSaturationLimit=Lower_saturation_limit
  Out1 : Outport
  wires:
  In1/1 -> Ki/1, Kp/1
  Kp/1 -> Sum12/2
  Ki/1 -> integrator/1
  integrator/1 -> Sum12/1
  Saturation2/1 -> Out1/1
  Sum12/1 -> Saturation2/1

== system M10B39_es_V1/Genrators/ES3/ control1/control_AC_voltage/Out_Q_Uac ==
  In1 : Inport
  Ki : Gain  Gain=KI_  SaturateOnIntegerOverflow=on  OutDataTypeStr=Inherit: Same as input  ParamDataTypeStr=Inherit: Same as input
  Kp : Gain  Gain=KP_  SaturateOnIntegerOverflow=on  OutDataTypeStr=Inherit: Same as input  ParamDataTypeStr=Inherit: Same as input
  Saturation2 : Saturate  UpperLimit=Upper_limit  LowerLimit=Lower_limit
  Sum12 : Sum  SaturateOnIntegerOverflow=on
  integrator : Integrator  InitialCondition=integrator_init  LimitOutput=on  UpperSaturationLimit=Upper_saturation_limit  LowerSaturationLimit=Lower_saturation_limit
  Out1 : Outport
  wires:
  In1/1 -> Ki/1, Kp/1
  Kp/1 -> Sum12/2
  Ki/1 -> integrator/1
  integrator/1 -> Sum12/1
  Saturation2/1 -> Out1/1
  Sum12/1 -> Saturation2/1

== system M10B39_es_V1/Genrators/ES3/ control1/control_AC_voltage1/Out_Q_Uac ==
  In1 : Inport
  Ki : Gain  Gain=KI_  SaturateOnIntegerOverflow=on  OutDataTypeStr=Inherit: Same as input  ParamDataTypeStr=Inherit: Same as input
  Kp : Gain  Gain=KP_  SaturateOnIntegerOverflow=on  OutDataTypeStr=Inherit: Same as input  ParamDataTypeStr=Inherit: Same as input
  Saturation2 : Saturate  UpperLimit=Upper_limit  LowerLimit=Lower_limit
  Sum12 : Sum  SaturateOnIntegerOverflow=on
  integrator : Integrator  InitialCondition=integrator_init  LimitOutput=on  UpperSaturationLimit=Upper_saturation_limit  LowerSaturationLimit=Lower_saturation_limit
  Out1 : Outport
  wires:
  In1/1 -> Ki/1, Kp/1
  Kp/1 -> Sum12/2
  Ki/1 -> integrator/1
  integrator/1 -> Sum12/1
  Saturation2/1 -> Out1/1
  Sum12/1 -> Saturation2/1
